simulink subsystem "MASS_PROPERTIES"  (R2025b)
settings: Solver=VariableStepAuto  StartTime=0.0  StopTime=10.0  RelTol=1e-3
model mask{dryMass=0, initFuelMass=0, dryInertia=0, fullInertia=0, inertiaBp=0, inertiaTab=0}
  mask prompts: dryMass "Dry mass [kg]"; initFuelMass "Initial fuel mass [kg]"; dryInertia "Dry inertia tensor [kgm2]"; fullInertia "Full inertia tensor [kgm2]"; inertiaBp "Inertia interpolation breakpoints"; inertiaTab "Inertia interpolation table"
undefined symbols (not defined in the file): simData
libraries: simulink_extras x1
settings Model: Creator=antoniohernandez-rodiciomateos  LastModifiedBy=antoniohernandez-rodiciomateos

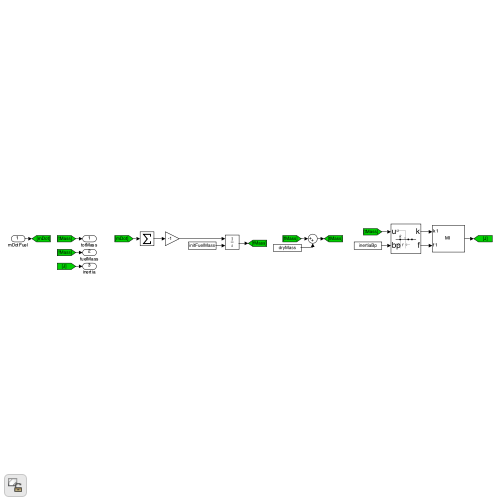
[thumbnail: Simulink's stored preview of the top-level diagram]
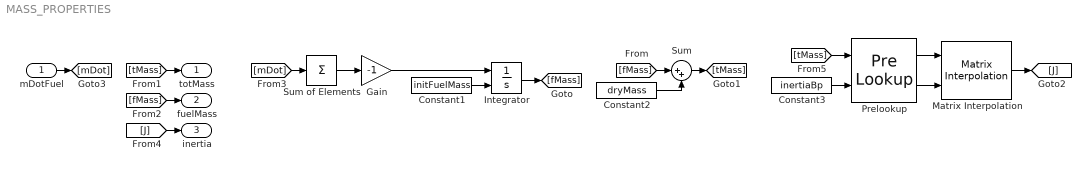
== system MASS_PROPERTIES ==
  mDotFuel : Inport  PortDimensions=[12 1]
  Constant1 : Constant  Value=initFuelMass
  Constant2 : Constant  Value=dryMass
  Constant3 : Constant  Value=inertiaBp
  Gain : Gain  Gain=-1
  Integrator : Integrator  InitialConditionSource=external
  Matrix Interpolation : simulink_extras/Additional Lookup Tables/Matrix Interpolation  InterpMethod=Linear  ExtrapMethod=Clip  InterpolateDimension=1  TableData=simData.massProperties.inertiaTab  SimulateUsing=Code generation
  Prelookup : PreLookup  BreakpointsDataSource=Input port  BreakpointsData=[10:10:110]  ExtrapMethod=Linear
      settings: InputPortMap=u0,p1
  Sum : Sum  Inputs=|++
  Sum of Elements : Sum  Inputs=+
  totMass : Outport  PortDimensions=[1 1]
  fuelMass : Outport  Port=2  PortDimensions=[1 1]
  inertia : Outport  Port=3  PortDimensions=[3 3]
  wires:
  Sum of Elements/1 -> Gain/1
  Gain/1 -> Integrator/1
  Constant1/1 -> Integrator/2
  Integrator/1 -> [fMass]
  [fMass] -> Sum/1
  Constant2/1 -> Sum/2
  Sum/1 -> [tMass]
  [fMass] -> fuelMass/1
  [tMass] -> totMass/1
  mDotFuel/1 -> [mDot]
  [mDot] -> Sum of Elements/1
  [J] -> inertia/1
  Constant3/1 -> Prelookup/2
  [tMass] -> Prelookup/1
  Prelookup/1 -> Matrix Interpolation/1
  Prelookup/2 -> Matrix Interpolation/2
  Matrix Interpolation/1 -> [J]
